simulink model "garage_door"  (R2018b)
settings: Solver=VariableStepAuto  StartTime=0.0  StopTime=10.0  RelTol=1e-3
libraries: simulink x1
settings Model: Creator=Filipowicz_user1  LastModifiedBy=jf

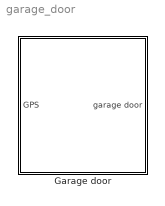
== system garage_door ==
  Garage door : Subsystem

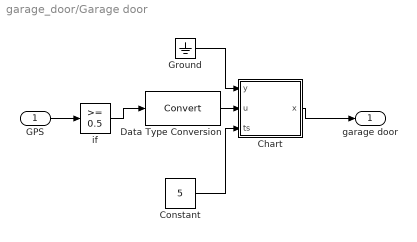
== system garage_door/Garage door ==
  GPS : Inport
  Chart : Stateflow chart  TreatAsAtomicUnit=on
  Constant : Constant  Value=5
  Data Type Conversion : DataTypeConversion
  Ground : Ground
  if : simulink/Logic and Bit Operations/Compare To Constant  relop=>=  const=0.5  OutDataTypeStr=boolean
  garage door : Outport
  wires:
  GPS/1 -> if/1
  Chart/1(x) -> garage door/1
  Constant/1 -> Chart/3(ts)
  Data Type Conversion/1 -> Chart/2(u)
  if/1 -> Data Type Conversion/1
  Ground/1 -> Chart/1(y)

== stateflow chart garage_door/Garage door/Chart ==
  settings: updateMethod=DISCRETE  sampleTime=1  executeAtInitialization=1
  state Idle
    x=0;
    t1=ts/timeStep;
  state State1
    x=1;
  state Wait
  (default) -> Idle
  Idle -> Idle [order 2]
  Wait -> Idle [order 2] : after(t1,'sec')
  Idle -> State1 [order 1] : [u>=1]
  State1 -> Idle [order 2] : [y==1]
  State1 -> Wait [order 1] : [u==0]
  Wait -> State1 [order 1] : [u==1]
  data: y input; u input; x output; ts input; timeStep constant double; t1 local
